simulink model "example"  (R2020a)
settings: Solver=VariableStepAuto  StartTime=0.0  StopTime=10.0  RelTol=1e-3
libraries: ros2lib x1

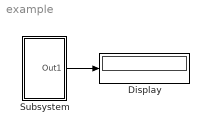
== system example ==
  Display : Display
  Subsystem : Subsystem
  wires:
  Subsystem/1(Out1) -> Display/1

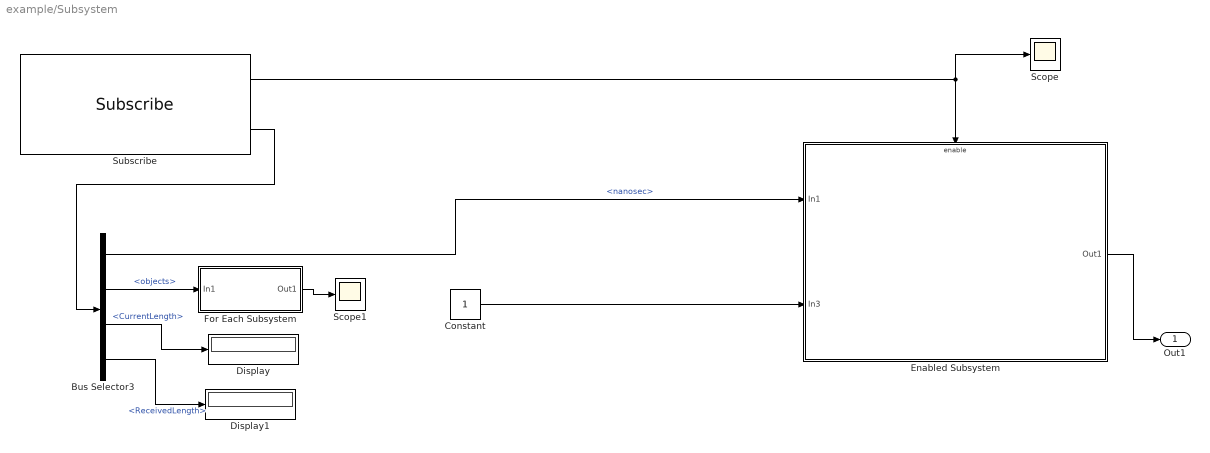
== system example/Subsystem ==
  Bus Selector3 : BusSelector  OutputSignals=header.stamp.nanosec,objects,objects_SL_Info.CurrentLength,objects_SL_Info.ReceivedLength
  Constant : Constant
  Display : Display
  Display1 : Display
  Enabled Subsystem : Subsystem  TreatAsAtomicUnit=on
  For Each Subsystem : Subsystem  TreatAsAtomicUnit=on
  Scope : Scope
  Scope1 : Scope
  Subscribe : ros2lib/Subscribe  topicSource=Specify your own  topic=/object_analytics/movement  messageType=object_analytics_msgs/MovingObjectsInFrame  sampleTime=-1  QOSHistory=Keep last  QOSDepth=1  QOSReliability=Reliable  QOSDurability=Volatile
      settings: SourceProductBaseCode=RR
  Out1 : Outport
  wires:
  Subscribe/2 -> Bus Selector3/1
  Enabled Subsystem/1(Out1) -> Out1/1
  Subscribe/1 -> Scope/1, Enabled Subsystem/Enable
  Bus Selector3/1 -> Enabled Subsystem/1(In1)  "<nanosec>"
  Bus Selector3/2 -> For Each Subsystem/1(In1)  "<objects>"
  Constant/1 -> Enabled Subsystem/2(In3)
  Bus Selector3/3 -> Display/1  "<CurrentLength>"
  Bus Selector3/4 -> Display1/1  "<ReceivedLength>"
  For Each Subsystem/1(Out1) -> Scope1/1

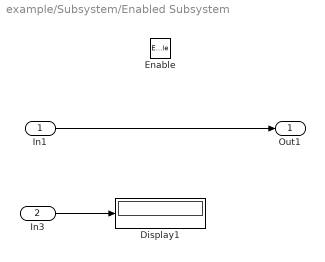
== system example/Subsystem/Enabled Subsystem ==
  In1 : Inport
  In3 : Inport  Port=2
  Enable : EnablePort
  Display1 : Display
  Out1 : Outport
  wires:
  In1/1 -> Out1/1
  In3/1 -> Display1/1

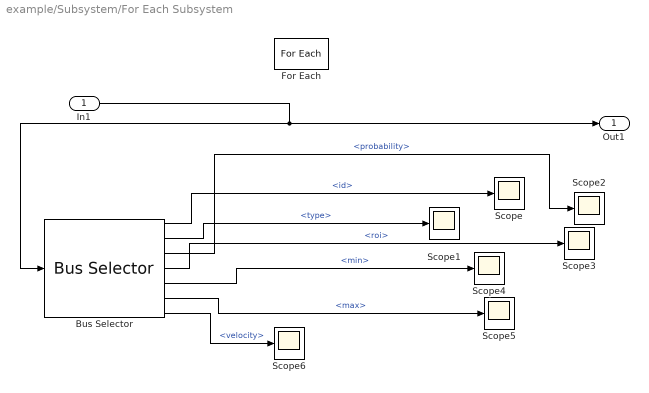
== system example/Subsystem/For Each Subsystem ==
  In1 : Inport  Partition=on  PartitionDimension=1  PartitionWidth=1  PartitionOffset=0
  Bus Selector : BusSelector  OutputSignals=id,type,probability,roi,min,max,velocity
  For Each : ForEach  DisableCoverage=on
  Scope{,1..6} (7 alike) : Scope
  Out1 : Outport  ConcatenationDimension=1
  wires:
  In1/1 -> Bus Selector/1, Out1/1
  Bus Selector/1 -> Scope/1  "<id>"
  Bus Selector/7 -> Scope6/1  "<velocity>"
  Bus Selector/2 -> Scope1/1  "<type>"
  Bus Selector/3 -> Scope2/1  "<probability>"
  Bus Selector/4 -> Scope3/1  "<roi>"
  Bus Selector/5 -> Scope4/1  "<min>"
  Bus Selector/6 -> Scope5/1  "<max>"
